simulink model "dinamicaralik"  (R2023b)
settings: Solver=ode45  StartTime=0.0  StopTime=50  FixedStep=0.0001  RelTol=1e-3
InitFcn:
  | Kpz = 0.3 ;
  | KIz = 0;
  | 
  | bh = 0.010290;  % batan hacim m^3
  | m = 10.5     ;  % aracın kütlesi kg
  | g = 9.81     ;  % yer çekimi ivmesi
  | p = 1000     ; % kg / m^3 yogunluk
  | W = m*g      ;  % aracın agırlıgı N
  | B = p*g*bh   ;  % Kaldırma kuvveti  N
  | 
  | xg = 0 ; % rgid body frame e göre ağırlık merkzi kordinatları
  | yg = 0 ;
  | zg = 0.02 ;
  | 
  | Ix = 0.1011 ; % kg *  m ^2
  | Iy = 0.1159 ;
  | Iz = 0.1615 ;
  | 
  | thrustCoefficient = 50/21.5 ;
  | 
  | % Add mass parametreleri
  | Xu_dot = -5.5;   % Surge direction
  | Yv_dot = -12.7;  % Sway direction
  | Zw_dot = -14.57; % Heave direction
  | 
  | Kp_dot = -0.12;  % Roll moment
  | Mq_dot = -0.12;  % Pitch moment
  | Nr_dot = -0.12;  % Yaw moment
  | 
  | % Linear Damping Values (Doğrusal Sönümleme Katsayıları)
  | Xu = -4.03;   % Ns/m
  | Yv = -6.22;   % Ns/m
  | Zw = -5.18;   % Ns/m
  | Kp = -0.07;   % Ns/rad
  | Mq = -0.07;   % Ns/rad
  | Nr = -0.07;   % Ns/rad
  | 
  | % Quadratic Damping Values (Doğrusal Olmayan Sönümleme Katsayıları)
  | Xuu = -18.18;  % Ns^2/m^2
  | Yvv = -21.66;  % Ns^2/m^2
  | Zww = -36.99;  % Ns^2/m^2
  | Kpp = -1.55;   % Ns^2/rad^2
  | Mqq = -1.55;   % Ns^2/rad^2
  | Nrr = -1.55;   % Ns^2/rad^2
undefined symbols (not defined in the file or in its folder): smiData, X, Y, Z
libraries: slpidlib x41, nesl_utility x14, sm_lib x12
(part 6 of 7)

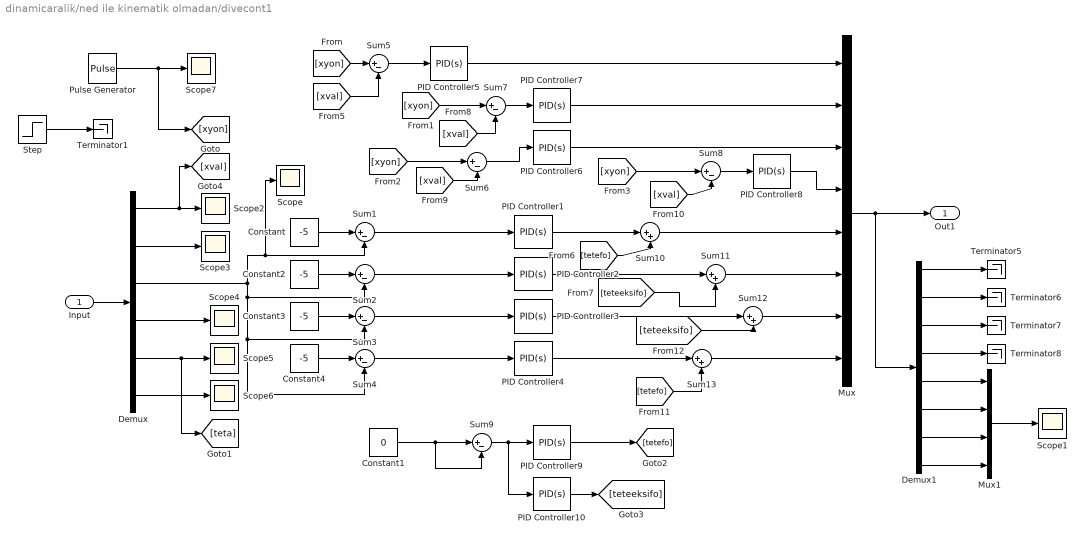
== system dinamicaralik/ned ile kinematik olmadan/divecont1 ==
  Input : Inport
  Constant{,2..4} (4 alike) : Constant  Value=-5
  Constant1 : Constant  Value=0
  Demux : Demux  Outputs=6
  Demux1 : Demux  Outputs=8
  Mux : Mux  Inputs=8
  Mux1 : Mux
  PID Controller1 : slpidlib/PID Controller  Controller=PID  Form=Parallel  TimeDomain=Continuous-time  UseExternalTs=off  SampleTime=-1  IntegratorMethod=Forward Euler  FilterMethod=Forward Euler  ControllerParametersSource=internal  P=Kpz  I=0  UseKiTs=off  D=0  N=100  UseFilter=on  TunerSelectOption=Transfer Function Based (PID Tuner App)  InitialConditionSource=internal  InitialConditionForIntegrator=0  InitialConditionForFilter=0  DifferentiatorICPrevScaledInput=0  ExternalReset=none  TrackingMode=off  Kt=1  LimitOutput=off  SatLimitsSource=internal  UpperSaturationLimit=inf  LowerSaturationLimit=-inf  LinearizeAsGain=on  AntiWindupMode=none  Kb=1  LimitIntegrator=off  UpperIntegratorSaturationLimit=inf  LowerIntegratorSaturationLimit=-inf  POutMin=[]  POutMax=[]  IOutMin=[]  IOutMax=[]  DOutMin=[]  DOutMax=[]  NOutMin=[]  NOutMax=[]  SumOutMin=[]  SumOutMax=[]  SaturationOutMin=[]  SaturationOutMax=[]  PParamMin=[]  PParamMax=[]  IParamMin=[]  IParamMax=[]  DParamMin=[]  DParamMax=[]  NParamMin=[]  NParamMax=[]  KbParamMin=[]  KbParamMax=[]  KtParamMin=[]  KtParamMax=[]  KbOutMin=[]  KbOutMax=[]  KtOutMin=[]  KtOutMax=[]  IntegratorOutMin=[]  IntegratorOutMax=[]  FilterOutMin=[]  FilterOutMax=[]  SumI1OutMin=[]  SumI1OutMax=[]  SumI2OutMin=[]  SumI2OutMax=[]  SumI3OutMin=[]  SumI3OutMax=[]  SumI4OutMin=[]  SumI4OutMax=[]  SumDOutMin=[]  SumDOutMax=[]  DifferentiatorOutMin=[]  DifferentiatorOutMax=[]  FilterDiffOutCoefMin=[]  FilterDiffOutCoefMax=[]  ReciprocalOutMin=[]  ReciprocalOutMax=[]  SumDenOutMin=[]  SumDenOutMax=[]  SumNumOutMin=[]  SumNumOutMax=[]  DivideOutMin=[]  DivideOutMax=[]  UdiffTsProdOutMin=[]  UdiffTsProdOutMax=[]  NTsProdOutMin=[]  NTsProdOutMax=[]  UintegralTsProdOutMin=[]  UintegralTsProdOutMax=[]  UngainTsProdOutMin=[]  UngainTsProdOutMax=[]  ClampingZeroOutDataTypeStr=Inherit: Inherit via back propagation  ClampingZeroOutMin=[]  ClampingZeroOutMax=[]  FilterDenConstantOutDataTypeStr=Inherit: Inherit via back propagation  FilterDenConstantOutMin=[]  FilterDenConstantOutMax=[]  PCopyOutDataTypeStr=Inherit: Inherit via back propagation  PCopyOutMin=[]  PCopyOutMax=[]  NCopyOutDataTypeStr=Inherit: Inherit via back propagation  NCopyOutMin=[]  NCopyOutMax=[]  IntegratorContinuousStateAttributes=''  IntegratorStateMustResolveToSignalObject=off  IntegratorRTWStateStorageClass=Auto  FilterContinuousStateAttributes=''  FilterStateMustResolveToSignalObject=off  FilterRTWStateStorageClass=Auto  ParallelPVariant=InternalParameters  IdealPVariant=Disabled  IVariant=InternalParameters  DVariant=InternalParameters  IntegratorVariant=Continuous  SatVariant=Disabled  AWVariant=Passthrough  PCopyVariant=Disabled  TRVariant=Disabled  FdbkBlocksVariant=Forward  IdealPFdbkVariant=Disabled  SatFdbkVariant=Disabled  DerivativeFilterVariant=ContFilter  NVariant=InternalParameters  NCopyVariant=Disabled  FilterICVariant=InternalICsFilter  IntegratorICVariant=InternalICs  ExternalResetVariant=Disabled  TRSumVariant=Passthrough  SumFdbkVariant=Disabled  SumVariant=Sum_PID  TsampFilterVariant=InternalTs  TsampNgainVariant=Passthrough  TsampIntegralVariant=Disabled_SignalSpec  ExternalSaturationOutDataTypeStr=Inherit: Same as second input
  PID Controller10 : slpidlib/PID Controller  Controller=PID  Form=Parallel  TimeDomain=Continuous-time  UseExternalTs=off  SampleTime=-1  IntegratorMethod=Forward Euler  FilterMethod=Forward Euler  ControllerParametersSource=internal  P=-0.1  I=0  UseKiTs=off  D=0  N=100  UseFilter=on  TunerSelectOption=Transfer Function Based (PID Tuner App)  InitialConditionSource=internal  InitialConditionForIntegrator=0  InitialConditionForFilter=0  DifferentiatorICPrevScaledInput=0  ExternalReset=none  TrackingMode=off  Kt=1  LimitOutput=off  SatLimitsSource=internal  UpperSaturationLimit=inf  LowerSaturationLimit=-inf  LinearizeAsGain=on  AntiWindupMode=none  Kb=1  LimitIntegrator=off  UpperIntegratorSaturationLimit=inf  LowerIntegratorSaturationLimit=-inf  POutMin=[]  POutMax=[]  IOutMin=[]  IOutMax=[]  DOutMin=[]  DOutMax=[]  NOutMin=[]  NOutMax=[]  SumOutMin=[]  SumOutMax=[]  SaturationOutMin=[]  SaturationOutMax=[]  PParamMin=[]  PParamMax=[]  IParamMin=[]  IParamMax=[]  DParamMin=[]  DParamMax=[]  NParamMin=[]  NParamMax=[]  KbParamMin=[]  KbParamMax=[]  KtParamMin=[]  KtParamMax=[]  KbOutMin=[]  KbOutMax=[]  KtOutMin=[]  KtOutMax=[]  IntegratorOutMin=[]  IntegratorOutMax=[]  FilterOutMin=[]  FilterOutMax=[]  SumI1OutMin=[]  SumI1OutMax=[]  SumI2OutMin=[]  SumI2OutMax=[]  SumI3OutMin=[]  SumI3OutMax=[]  SumI4OutMin=[]  SumI4OutMax=[]  SumDOutMin=[]  SumDOutMax=[]  DifferentiatorOutMin=[]  DifferentiatorOutMax=[]  FilterDiffOutCoefMin=[]  FilterDiffOutCoefMax=[]  ReciprocalOutMin=[]  ReciprocalOutMax=[]  SumDenOutMin=[]  SumDenOutMax=[]  SumNumOutMin=[]  SumNumOutMax=[]  DivideOutMin=[]  DivideOutMax=[]  UdiffTsProdOutMin=[]  UdiffTsProdOutMax=[]  NTsProdOutMin=[]  NTsProdOutMax=[]  UintegralTsProdOutMin=[]  UintegralTsProdOutMax=[]  UngainTsProdOutMin=[]  UngainTsProdOutMax=[]  ClampingZeroOutDataTypeStr=Inherit: Inherit via back propagation  ClampingZeroOutMin=[]  ClampingZeroOutMax=[]  FilterDenConstantOutDataTypeStr=Inherit: Inherit via back propagation  FilterDenConstantOutMin=[]  FilterDenConstantOutMax=[]  PCopyOutDataTypeStr=Inherit: Inherit via back propagation  PCopyOutMin=[]  PCopyOutMax=[]  NCopyOutDataTypeStr=Inherit: Inherit via back propagation  NCopyOutMin=[]  NCopyOutMax=[]  IntegratorContinuousStateAttributes=''  IntegratorStateMustResolveToSignalObject=off  IntegratorRTWStateStorageClass=Auto  FilterContinuousStateAttributes=''  FilterStateMustResolveToSignalObject=off  FilterRTWStateStorageClass=Auto  ParallelPVariant=InternalParameters  IdealPVariant=Disabled  IVariant=InternalParameters  DVariant=InternalParameters  IntegratorVariant=Continuous  SatVariant=Disabled  AWVariant=Passthrough  PCopyVariant=Disabled  TRVariant=Disabled  FdbkBlocksVariant=Forward  IdealPFdbkVariant=Disabled  SatFdbkVariant=Disabled  DerivativeFilterVariant=ContFilter  NVariant=InternalParameters  NCopyVariant=Disabled  FilterICVariant=InternalICsFilter  IntegratorICVariant=InternalICs  ExternalResetVariant=Disabled  TRSumVariant=Passthrough  SumFdbkVariant=Disabled  SumVariant=Sum_PID  TsampFilterVariant=InternalTs  TsampNgainVariant=Passthrough  TsampIntegralVariant=Disabled_SignalSpec  ExternalSaturationOutDataTypeStr=Inherit: Same as second input
  PID Controller2 : slpidlib/PID Controller  Controller=PID  Form=Parallel  TimeDomain=Continuous-time  UseExternalTs=off  SampleTime=-1  IntegratorMethod=Forward Euler  FilterMethod=Forward Euler  ControllerParametersSource=internal  P=-Kpz  I=0  UseKiTs=off  D=0  N=100  UseFilter=on  TunerSelectOption=Transfer Function Based (PID Tuner App)  InitialConditionSource=internal  InitialConditionForIntegrator=0  InitialConditionForFilter=0  DifferentiatorICPrevScaledInput=0  ExternalReset=none  TrackingMode=off  Kt=1  LimitOutput=off  SatLimitsSource=internal  UpperSaturationLimit=inf  LowerSaturationLimit=-inf  LinearizeAsGain=on  AntiWindupMode=none  Kb=1  LimitIntegrator=off  UpperIntegratorSaturationLimit=inf  LowerIntegratorSaturationLimit=-inf  POutMin=[]  POutMax=[]  IOutMin=[]  IOutMax=[]  DOutMin=[]  DOutMax=[]  NOutMin=[]  NOutMax=[]  SumOutMin=[]  SumOutMax=[]  SaturationOutMin=[]  SaturationOutMax=[]  PParamMin=[]  PParamMax=[]  IParamMin=[]  IParamMax=[]  DParamMin=[]  DParamMax=[]  NParamMin=[]  NParamMax=[]  KbParamMin=[]  KbParamMax=[]  KtParamMin=[]  KtParamMax=[]  KbOutMin=[]  KbOutMax=[]  KtOutMin=[]  KtOutMax=[]  IntegratorOutMin=[]  IntegratorOutMax=[]  FilterOutMin=[]  FilterOutMax=[]  SumI1OutMin=[]  SumI1OutMax=[]  SumI2OutMin=[]  SumI2OutMax=[]  SumI3OutMin=[]  SumI3OutMax=[]  SumI4OutMin=[]  SumI4OutMax=[]  SumDOutMin=[]  SumDOutMax=[]  DifferentiatorOutMin=[]  DifferentiatorOutMax=[]  FilterDiffOutCoefMin=[]  FilterDiffOutCoefMax=[]  ReciprocalOutMin=[]  ReciprocalOutMax=[]  SumDenOutMin=[]  SumDenOutMax=[]  SumNumOutMin=[]  SumNumOutMax=[]  DivideOutMin=[]  DivideOutMax=[]  UdiffTsProdOutMin=[]  UdiffTsProdOutMax=[]  NTsProdOutMin=[]  NTsProdOutMax=[]  UintegralTsProdOutMin=[]  UintegralTsProdOutMax=[]  UngainTsProdOutMin=[]  UngainTsProdOutMax=[]  ClampingZeroOutDataTypeStr=Inherit: Inherit via back propagation  ClampingZeroOutMin=[]  ClampingZeroOutMax=[]  FilterDenConstantOutDataTypeStr=Inherit: Inherit via back propagation  FilterDenConstantOutMin=[]  FilterDenConstantOutMax=[]  PCopyOutDataTypeStr=Inherit: Inherit via back propagation  PCopyOutMin=[]  PCopyOutMax=[]  NCopyOutDataTypeStr=Inherit: Inherit via back propagation  NCopyOutMin=[]  NCopyOutMax=[]  IntegratorContinuousStateAttributes=''  IntegratorStateMustResolveToSignalObject=off  IntegratorRTWStateStorageClass=Auto  FilterContinuousStateAttributes=''  FilterStateMustResolveToSignalObject=off  FilterRTWStateStorageClass=Auto  ParallelPVariant=InternalParameters  IdealPVariant=Disabled  IVariant=InternalParameters  DVariant=InternalParameters  IntegratorVariant=Continuous  SatVariant=Disabled  AWVariant=Passthrough  PCopyVariant=Disabled  TRVariant=Disabled  FdbkBlocksVariant=Forward  IdealPFdbkVariant=Disabled  SatFdbkVariant=Disabled  DerivativeFilterVariant=ContFilter  NVariant=InternalParameters  NCopyVariant=Disabled  FilterICVariant=InternalICsFilter  IntegratorICVariant=InternalICs  ExternalResetVariant=Disabled  TRSumVariant=Passthrough  SumFdbkVariant=Disabled  SumVariant=Sum_PID  TsampFilterVariant=InternalTs  TsampNgainVariant=Passthrough  TsampIntegralVariant=Disabled_SignalSpec  ExternalSaturationOutDataTypeStr=Inherit: Same as second input
  PID Controller3 : slpidlib/PID Controller  Controller=PID  Form=Parallel  TimeDomain=Continuous-time  UseExternalTs=off  SampleTime=-1  IntegratorMethod=Forward Euler  FilterMethod=Forward Euler  ControllerParametersSource=internal  P=-Kpz  I=0  UseKiTs=off  D=0  N=100  UseFilter=on  TunerSelectOption=Transfer Function Based (PID Tuner App)  InitialConditionSource=internal  InitialConditionForIntegrator=0  InitialConditionForFilter=0  DifferentiatorICPrevScaledInput=0  ExternalReset=none  TrackingMode=off  Kt=1  LimitOutput=off  SatLimitsSource=internal  UpperSaturationLimit=inf  LowerSaturationLimit=-inf  LinearizeAsGain=on  AntiWindupMode=none  Kb=1  LimitIntegrator=off  UpperIntegratorSaturationLimit=inf  LowerIntegratorSaturationLimit=-inf  POutMin=[]  POutMax=[]  IOutMin=[]  IOutMax=[]  DOutMin=[]  DOutMax=[]  NOutMin=[]  NOutMax=[]  SumOutMin=[]  SumOutMax=[]  SaturationOutMin=[]  SaturationOutMax=[]  PParamMin=[]  PParamMax=[]  IParamMin=[]  IParamMax=[]  DParamMin=[]  DParamMax=[]  NParamMin=[]  NParamMax=[]  KbParamMin=[]  KbParamMax=[]  KtParamMin=[]  KtParamMax=[]  KbOutMin=[]  KbOutMax=[]  KtOutMin=[]  KtOutMax=[]  IntegratorOutMin=[]  IntegratorOutMax=[]  FilterOutMin=[]  FilterOutMax=[]  SumI1OutMin=[]  SumI1OutMax=[]  SumI2OutMin=[]  SumI2OutMax=[]  SumI3OutMin=[]  SumI3OutMax=[]  SumI4OutMin=[]  SumI4OutMax=[]  SumDOutMin=[]  SumDOutMax=[]  DifferentiatorOutMin=[]  DifferentiatorOutMax=[]  FilterDiffOutCoefMin=[]  FilterDiffOutCoefMax=[]  ReciprocalOutMin=[]  ReciprocalOutMax=[]  SumDenOutMin=[]  SumDenOutMax=[]  SumNumOutMin=[]  SumNumOutMax=[]  DivideOutMin=[]  DivideOutMax=[]  UdiffTsProdOutMin=[]  UdiffTsProdOutMax=[]  NTsProdOutMin=[]  NTsProdOutMax=[]  UintegralTsProdOutMin=[]  UintegralTsProdOutMax=[]  UngainTsProdOutMin=[]  UngainTsProdOutMax=[]  ClampingZeroOutDataTypeStr=Inherit: Inherit via back propagation  ClampingZeroOutMin=[]  ClampingZeroOutMax=[]  FilterDenConstantOutDataTypeStr=Inherit: Inherit via back propagation  FilterDenConstantOutMin=[]  FilterDenConstantOutMax=[]  PCopyOutDataTypeStr=Inherit: Inherit via back propagation  PCopyOutMin=[]  PCopyOutMax=[]  NCopyOutDataTypeStr=Inherit: Inherit via back propagation  NCopyOutMin=[]  NCopyOutMax=[]  IntegratorContinuousStateAttributes=''  IntegratorStateMustResolveToSignalObject=off  IntegratorRTWStateStorageClass=Auto  FilterContinuousStateAttributes=''  FilterStateMustResolveToSignalObject=off  FilterRTWStateStorageClass=Auto  ParallelPVariant=InternalParameters  IdealPVariant=Disabled  IVariant=InternalParameters  DVariant=InternalParameters  IntegratorVariant=Continuous  SatVariant=Disabled  AWVariant=Passthrough  PCopyVariant=Disabled  TRVariant=Disabled  FdbkBlocksVariant=Forward  IdealPFdbkVariant=Disabled  SatFdbkVariant=Disabled  DerivativeFilterVariant=ContFilter  NVariant=InternalParameters  NCopyVariant=Disabled  FilterICVariant=InternalICsFilter  IntegratorICVariant=InternalICs  ExternalResetVariant=Disabled  TRSumVariant=Passthrough  SumFdbkVariant=Disabled  SumVariant=Sum_PID  TsampFilterVariant=InternalTs  TsampNgainVariant=Passthrough  TsampIntegralVariant=Disabled_SignalSpec  ExternalSaturationOutDataTypeStr=Inherit: Same as second input
  PID Controller4 : slpidlib/PID Controller  Controller=PID  Form=Parallel  TimeDomain=Continuous-time  UseExternalTs=off  SampleTime=-1  IntegratorMethod=Forward Euler  FilterMethod=Forward Euler  ControllerParametersSource=internal  P=Kpz  I=0  UseKiTs=off  D=0  N=100  UseFilter=on  TunerSelectOption=Transfer Function Based (PID Tuner App)  InitialConditionSource=internal  InitialConditionForIntegrator=0  InitialConditionForFilter=0  DifferentiatorICPrevScaledInput=0  ExternalReset=none  TrackingMode=off  Kt=1  LimitOutput=off  SatLimitsSource=internal  UpperSaturationLimit=inf  LowerSaturationLimit=-inf  LinearizeAsGain=on  AntiWindupMode=none  Kb=1  LimitIntegrator=off  UpperIntegratorSaturationLimit=inf  LowerIntegratorSaturationLimit=-inf  POutMin=[]  POutMax=[]  IOutMin=[]  IOutMax=[]  DOutMin=[]  DOutMax=[]  NOutMin=[]  NOutMax=[]  SumOutMin=[]  SumOutMax=[]  SaturationOutMin=[]  SaturationOutMax=[]  PParamMin=[]  PParamMax=[]  IParamMin=[]  IParamMax=[]  DParamMin=[]  DParamMax=[]  NParamMin=[]  NParamMax=[]  KbParamMin=[]  KbParamMax=[]  KtParamMin=[]  KtParamMax=[]  KbOutMin=[]  KbOutMax=[]  KtOutMin=[]  KtOutMax=[]  IntegratorOutMin=[]  IntegratorOutMax=[]  FilterOutMin=[]  FilterOutMax=[]  SumI1OutMin=[]  SumI1OutMax=[]  SumI2OutMin=[]  SumI2OutMax=[]  SumI3OutMin=[]  SumI3OutMax=[]  SumI4OutMin=[]  SumI4OutMax=[]  SumDOutMin=[]  SumDOutMax=[]  DifferentiatorOutMin=[]  DifferentiatorOutMax=[]  FilterDiffOutCoefMin=[]  FilterDiffOutCoefMax=[]  ReciprocalOutMin=[]  ReciprocalOutMax=[]  SumDenOutMin=[]  SumDenOutMax=[]  SumNumOutMin=[]  SumNumOutMax=[]  DivideOutMin=[]  DivideOutMax=[]  UdiffTsProdOutMin=[]  UdiffTsProdOutMax=[]  NTsProdOutMin=[]  NTsProdOutMax=[]  UintegralTsProdOutMin=[]  UintegralTsProdOutMax=[]  UngainTsProdOutMin=[]  UngainTsProdOutMax=[]  ClampingZeroOutDataTypeStr=Inherit: Inherit via back propagation  ClampingZeroOutMin=[]  ClampingZeroOutMax=[]  FilterDenConstantOutDataTypeStr=Inherit: Inherit via back propagation  FilterDenConstantOutMin=[]  FilterDenConstantOutMax=[]  PCopyOutDataTypeStr=Inherit: Inherit via back propagation  PCopyOutMin=[]  PCopyOutMax=[]  NCopyOutDataTypeStr=Inherit: Inherit via back propagation  NCopyOutMin=[]  NCopyOutMax=[]  IntegratorContinuousStateAttributes=''  IntegratorStateMustResolveToSignalObject=off  IntegratorRTWStateStorageClass=Auto  FilterContinuousStateAttributes=''  FilterStateMustResolveToSignalObject=off  FilterRTWStateStorageClass=Auto  ParallelPVariant=InternalParameters  IdealPVariant=Disabled  IVariant=InternalParameters  DVariant=InternalParameters  IntegratorVariant=Continuous  SatVariant=Disabled  AWVariant=Passthrough  PCopyVariant=Disabled  TRVariant=Disabled  FdbkBlocksVariant=Forward  IdealPFdbkVariant=Disabled  SatFdbkVariant=Disabled  DerivativeFilterVariant=ContFilter  NVariant=InternalParameters  NCopyVariant=Disabled  FilterICVariant=InternalICsFilter  IntegratorICVariant=InternalICs  ExternalResetVariant=Disabled  TRSumVariant=Passthrough  SumFdbkVariant=Disabled  SumVariant=Sum_PID  TsampFilterVariant=InternalTs  TsampNgainVariant=Passthrough  TsampIntegralVariant=Disabled_SignalSpec  ExternalSaturationOutDataTypeStr=Inherit: Same as second input
  PID Controller5 : slpidlib/PID Controller  Controller=PID  Form=Parallel  TimeDomain=Continuous-time  UseExternalTs=off  SampleTime=-1  IntegratorMethod=Forward Euler  FilterMethod=Forward Euler  ControllerParametersSource=internal  P=Kpz  I=KIz  UseKiTs=off  D=0  N=100  UseFilter=on  TunerSelectOption=Transfer Function Based (PID Tuner App)  InitialConditionSource=internal  InitialConditionForIntegrator=0  InitialConditionForFilter=0  DifferentiatorICPrevScaledInput=0  ExternalReset=none  TrackingMode=off  Kt=1  LimitOutput=off  SatLimitsSource=internal  UpperSaturationLimit=inf  LowerSaturationLimit=-inf  LinearizeAsGain=on  AntiWindupMode=none  Kb=1  LimitIntegrator=off  UpperIntegratorSaturationLimit=inf  LowerIntegratorSaturationLimit=-inf  POutMin=[]  POutMax=[]  IOutMin=[]  IOutMax=[]  DOutMin=[]  DOutMax=[]  NOutMin=[]  NOutMax=[]  SumOutMin=[]  SumOutMax=[]  SaturationOutMin=[]  SaturationOutMax=[]  PParamMin=[]  PParamMax=[]  IParamMin=[]  IParamMax=[]  DParamMin=[]  DParamMax=[]  NParamMin=[]  NParamMax=[]  KbParamMin=[]  KbParamMax=[]  KtParamMin=[]  KtParamMax=[]  KbOutMin=[]  KbOutMax=[]  KtOutMin=[]  KtOutMax=[]  IntegratorOutMin=[]  IntegratorOutMax=[]  FilterOutMin=[]  FilterOutMax=[]  SumI1OutMin=[]  SumI1OutMax=[]  SumI2OutMin=[]  SumI2OutMax=[]  SumI3OutMin=[]  SumI3OutMax=[]  SumI4OutMin=[]  SumI4OutMax=[]  SumDOutMin=[]  SumDOutMax=[]  DifferentiatorOutMin=[]  DifferentiatorOutMax=[]  FilterDiffOutCoefMin=[]  FilterDiffOutCoefMax=[]  ReciprocalOutMin=[]  ReciprocalOutMax=[]  SumDenOutMin=[]  SumDenOutMax=[]  SumNumOutMin=[]  SumNumOutMax=[]  DivideOutMin=[]  DivideOutMax=[]  UdiffTsProdOutMin=[]  UdiffTsProdOutMax=[]  NTsProdOutMin=[]  NTsProdOutMax=[]  UintegralTsProdOutMin=[]  UintegralTsProdOutMax=[]  UngainTsProdOutMin=[]  UngainTsProdOutMax=[]  ClampingZeroOutDataTypeStr=Inherit: Inherit via back propagation  ClampingZeroOutMin=[]  ClampingZeroOutMax=[]  FilterDenConstantOutDataTypeStr=Inherit: Inherit via back propagation  FilterDenConstantOutMin=[]  FilterDenConstantOutMax=[]  PCopyOutDataTypeStr=Inherit: Inherit via back propagation  PCopyOutMin=[]  PCopyOutMax=[]  NCopyOutDataTypeStr=Inherit: Inherit via back propagation  NCopyOutMin=[]  NCopyOutMax=[]  IntegratorContinuousStateAttributes=''  IntegratorStateMustResolveToSignalObject=off  IntegratorRTWStateStorageClass=Auto  FilterContinuousStateAttributes=''  FilterStateMustResolveToSignalObject=off  FilterRTWStateStorageClass=Auto  ParallelPVariant=InternalParameters  IdealPVariant=Disabled  IVariant=InternalParameters  DVariant=InternalParameters  IntegratorVariant=Continuous  SatVariant=Disabled  AWVariant=Passthrough  PCopyVariant=Disabled  TRVariant=Disabled  FdbkBlocksVariant=Forward  IdealPFdbkVariant=Disabled  SatFdbkVariant=Disabled  DerivativeFilterVariant=ContFilter  NVariant=InternalParameters  NCopyVariant=Disabled  FilterICVariant=InternalICsFilter  IntegratorICVariant=InternalICs  ExternalResetVariant=Disabled  TRSumVariant=Passthrough  SumFdbkVariant=Disabled  SumVariant=Sum_PID  TsampFilterVariant=InternalTs  TsampNgainVariant=Passthrough  TsampIntegralVariant=Disabled_SignalSpec  ExternalSaturationOutDataTypeStr=Inherit: Same as second input
  PID Controller6 : slpidlib/PID Controller  Controller=PID  Form=Parallel  TimeDomain=Continuous-time  UseExternalTs=off  SampleTime=-1  IntegratorMethod=Forward Euler  FilterMethod=Forward Euler  ControllerParametersSource=internal  P=-Kpz  I=KIz  UseKiTs=off  D=0  N=100  UseFilter=on  TunerSelectOption=Transfer Function Based (PID Tuner App)  InitialConditionSource=internal  InitialConditionForIntegrator=0  InitialConditionForFilter=0  DifferentiatorICPrevScaledInput=0  ExternalReset=none  TrackingMode=off  Kt=1  LimitOutput=off  SatLimitsSource=internal  UpperSaturationLimit=inf  LowerSaturationLimit=-inf  LinearizeAsGain=on  AntiWindupMode=none  Kb=1  LimitIntegrator=off  UpperIntegratorSaturationLimit=inf  LowerIntegratorSaturationLimit=-inf  POutMin=[]  POutMax=[]  IOutMin=[]  IOutMax=[]  DOutMin=[]  DOutMax=[]  NOutMin=[]  NOutMax=[]  SumOutMin=[]  SumOutMax=[]  SaturationOutMin=[]  SaturationOutMax=[]  PParamMin=[]  PParamMax=[]  IParamMin=[]  IParamMax=[]  DParamMin=[]  DParamMax=[]  NParamMin=[]  NParamMax=[]  KbParamMin=[]  KbParamMax=[]  KtParamMin=[]  KtParamMax=[]  KbOutMin=[]  KbOutMax=[]  KtOutMin=[]  KtOutMax=[]  IntegratorOutMin=[]  IntegratorOutMax=[]  FilterOutMin=[]  FilterOutMax=[]  SumI1OutMin=[]  SumI1OutMax=[]  SumI2OutMin=[]  SumI2OutMax=[]  SumI3OutMin=[]  SumI3OutMax=[]  SumI4OutMin=[]  SumI4OutMax=[]  SumDOutMin=[]  SumDOutMax=[]  DifferentiatorOutMin=[]  DifferentiatorOutMax=[]  FilterDiffOutCoefMin=[]  FilterDiffOutCoefMax=[]  ReciprocalOutMin=[]  ReciprocalOutMax=[]  SumDenOutMin=[]  SumDenOutMax=[]  SumNumOutMin=[]  SumNumOutMax=[]  DivideOutMin=[]  DivideOutMax=[]  UdiffTsProdOutMin=[]  UdiffTsProdOutMax=[]  NTsProdOutMin=[]  NTsProdOutMax=[]  UintegralTsProdOutMin=[]  UintegralTsProdOutMax=[]  UngainTsProdOutMin=[]  UngainTsProdOutMax=[]  ClampingZeroOutDataTypeStr=Inherit: Inherit via back propagation  ClampingZeroOutMin=[]  ClampingZeroOutMax=[]  FilterDenConstantOutDataTypeStr=Inherit: Inherit via back propagation  FilterDenConstantOutMin=[]  FilterDenConstantOutMax=[]  PCopyOutDataTypeStr=Inherit: Inherit via back propagation  PCopyOutMin=[]  PCopyOutMax=[]  NCopyOutDataTypeStr=Inherit: Inherit via back propagation  NCopyOutMin=[]  NCopyOutMax=[]  IntegratorContinuousStateAttributes=''  IntegratorStateMustResolveToSignalObject=off  IntegratorRTWStateStorageClass=Auto  FilterContinuousStateAttributes=''  FilterStateMustResolveToSignalObject=off  FilterRTWStateStorageClass=Auto  ParallelPVariant=InternalParameters  IdealPVariant=Disabled  IVariant=InternalParameters  DVariant=InternalParameters  IntegratorVariant=Continuous  SatVariant=Disabled  AWVariant=Passthrough  PCopyVariant=Disabled  TRVariant=Disabled  FdbkBlocksVariant=Forward  IdealPFdbkVariant=Disabled  SatFdbkVariant=Disabled  DerivativeFilterVariant=ContFilter  NVariant=InternalParameters  NCopyVariant=Disabled  FilterICVariant=InternalICsFilter  IntegratorICVariant=InternalICs  ExternalResetVariant=Disabled  TRSumVariant=Passthrough  SumFdbkVariant=Disabled  SumVariant=Sum_PID  TsampFilterVariant=InternalTs  TsampNgainVariant=Passthrough  TsampIntegralVariant=Disabled_SignalSpec  ExternalSaturationOutDataTypeStr=Inherit: Same as second input
  PID Controller7 : slpidlib/PID Controller  Controller=PID  Form=Parallel  TimeDomain=Continuous-time  UseExternalTs=off  SampleTime=-1  IntegratorMethod=Forward Euler  FilterMethod=Forward Euler  ControllerParametersSource=internal  P=Kpz  I=KIz  UseKiTs=off  D=0  N=100  UseFilter=on  TunerSelectOption=Transfer Function Based (PID Tuner App)  InitialConditionSource=internal  InitialConditionForIntegrator=0  InitialConditionForFilter=0  DifferentiatorICPrevScaledInput=0  ExternalReset=none  TrackingMode=off  Kt=1  LimitOutput=off  SatLimitsSource=internal  UpperSaturationLimit=inf  LowerSaturationLimit=-inf  LinearizeAsGain=on  AntiWindupMode=none  Kb=1  LimitIntegrator=off  UpperIntegratorSaturationLimit=inf  LowerIntegratorSaturationLimit=-inf  POutMin=[]  POutMax=[]  IOutMin=[]  IOutMax=[]  DOutMin=[]  DOutMax=[]  NOutMin=[]  NOutMax=[]  SumOutMin=[]  SumOutMax=[]  SaturationOutMin=[]  SaturationOutMax=[]  PParamMin=[]  PParamMax=[]  IParamMin=[]  IParamMax=[]  DParamMin=[]  DParamMax=[]  NParamMin=[]  NParamMax=[]  KbParamMin=[]  KbParamMax=[]  KtParamMin=[]  KtParamMax=[]  KbOutMin=[]  KbOutMax=[]  KtOutMin=[]  KtOutMax=[]  IntegratorOutMin=[]  IntegratorOutMax=[]  FilterOutMin=[]  FilterOutMax=[]  SumI1OutMin=[]  SumI1OutMax=[]  SumI2OutMin=[]  SumI2OutMax=[]  SumI3OutMin=[]  SumI3OutMax=[]  SumI4OutMin=[]  SumI4OutMax=[]  SumDOutMin=[]  SumDOutMax=[]  DifferentiatorOutMin=[]  DifferentiatorOutMax=[]  FilterDiffOutCoefMin=[]  FilterDiffOutCoefMax=[]  ReciprocalOutMin=[]  ReciprocalOutMax=[]  SumDenOutMin=[]  SumDenOutMax=[]  SumNumOutMin=[]  SumNumOutMax=[]  DivideOutMin=[]  DivideOutMax=[]  UdiffTsProdOutMin=[]  UdiffTsProdOutMax=[]  NTsProdOutMin=[]  NTsProdOutMax=[]  UintegralTsProdOutMin=[]  UintegralTsProdOutMax=[]  UngainTsProdOutMin=[]  UngainTsProdOutMax=[]  ClampingZeroOutDataTypeStr=Inherit: Inherit via back propagation  ClampingZeroOutMin=[]  ClampingZeroOutMax=[]  FilterDenConstantOutDataTypeStr=Inherit: Inherit via back propagation  FilterDenConstantOutMin=[]  FilterDenConstantOutMax=[]  PCopyOutDataTypeStr=Inherit: Inherit via back propagation  PCopyOutMin=[]  PCopyOutMax=[]  NCopyOutDataTypeStr=Inherit: Inherit via back propagation  NCopyOutMin=[]  NCopyOutMax=[]  IntegratorContinuousStateAttributes=''  IntegratorStateMustResolveToSignalObject=off  IntegratorRTWStateStorageClass=Auto  FilterContinuousStateAttributes=''  FilterStateMustResolveToSignalObject=off  FilterRTWStateStorageClass=Auto  ParallelPVariant=InternalParameters  IdealPVariant=Disabled  IVariant=InternalParameters  DVariant=InternalParameters  IntegratorVariant=Continuous  SatVariant=Disabled  AWVariant=Passthrough  PCopyVariant=Disabled  TRVariant=Disabled  FdbkBlocksVariant=Forward  IdealPFdbkVariant=Disabled  SatFdbkVariant=Disabled  DerivativeFilterVariant=ContFilter  NVariant=InternalParameters  NCopyVariant=Disabled  FilterICVariant=InternalICsFilter  IntegratorICVariant=InternalICs  ExternalResetVariant=Disabled  TRSumVariant=Passthrough  SumFdbkVariant=Disabled  SumVariant=Sum_PID  TsampFilterVariant=InternalTs  TsampNgainVariant=Passthrough  TsampIntegralVariant=Disabled_SignalSpec  ExternalSaturationOutDataTypeStr=Inherit: Same as second input
  PID Controller8 : slpidlib/PID Controller  Controller=PID  Form=Parallel  TimeDomain=Continuous-time  UseExternalTs=off  SampleTime=-1  IntegratorMethod=Forward Euler  FilterMethod=Forward Euler  ControllerParametersSource=internal  P=-Kpz  I=KIz  UseKiTs=off  D=0  N=100  UseFilter=on  TunerSelectOption=Transfer Function Based (PID Tuner App)  InitialConditionSource=internal  InitialConditionForIntegrator=0  InitialConditionForFilter=0  DifferentiatorICPrevScaledInput=0  ExternalReset=none  TrackingMode=off  Kt=1  LimitOutput=off  SatLimitsSource=internal  UpperSaturationLimit=inf  LowerSaturationLimit=-inf  LinearizeAsGain=on  AntiWindupMode=none  Kb=1  LimitIntegrator=off  UpperIntegratorSaturationLimit=inf  LowerIntegratorSaturationLimit=-inf  POutMin=[]  POutMax=[]  IOutMin=[]  IOutMax=[]  DOutMin=[]  DOutMax=[]  NOutMin=[]  NOutMax=[]  SumOutMin=[]  SumOutMax=[]  SaturationOutMin=[]  SaturationOutMax=[]  PParamMin=[]  PParamMax=[]  IParamMin=[]  IParamMax=[]  DParamMin=[]  DParamMax=[]  NParamMin=[]  NParamMax=[]  KbParamMin=[]  KbParamMax=[]  KtParamMin=[]  KtParamMax=[]  KbOutMin=[]  KbOutMax=[]  KtOutMin=[]  KtOutMax=[]  IntegratorOutMin=[]  IntegratorOutMax=[]  FilterOutMin=[]  FilterOutMax=[]  SumI1OutMin=[]  SumI1OutMax=[]  SumI2OutMin=[]  SumI2OutMax=[]  SumI3OutMin=[]  SumI3OutMax=[]  SumI4OutMin=[]  SumI4OutMax=[]  SumDOutMin=[]  SumDOutMax=[]  DifferentiatorOutMin=[]  DifferentiatorOutMax=[]  FilterDiffOutCoefMin=[]  FilterDiffOutCoefMax=[]  ReciprocalOutMin=[]  ReciprocalOutMax=[]  SumDenOutMin=[]  SumDenOutMax=[]  SumNumOutMin=[]  SumNumOutMax=[]  DivideOutMin=[]  DivideOutMax=[]  UdiffTsProdOutMin=[]  UdiffTsProdOutMax=[]  NTsProdOutMin=[]  NTsProdOutMax=[]  UintegralTsProdOutMin=[]  UintegralTsProdOutMax=[]  UngainTsProdOutMin=[]  UngainTsProdOutMax=[]  ClampingZeroOutDataTypeStr=Inherit: Inherit via back propagation  ClampingZeroOutMin=[]  ClampingZeroOutMax=[]  FilterDenConstantOutDataTypeStr=Inherit: Inherit via back propagation  FilterDenConstantOutMin=[]  FilterDenConstantOutMax=[]  PCopyOutDataTypeStr=Inherit: Inherit via back propagation  PCopyOutMin=[]  PCopyOutMax=[]  NCopyOutDataTypeStr=Inherit: Inherit via back propagation  NCopyOutMin=[]  NCopyOutMax=[]  IntegratorContinuousStateAttributes=''  IntegratorStateMustResolveToSignalObject=off  IntegratorRTWStateStorageClass=Auto  FilterContinuousStateAttributes=''  FilterStateMustResolveToSignalObject=off  FilterRTWStateStorageClass=Auto  ParallelPVariant=InternalParameters  IdealPVariant=Disabled  IVariant=InternalParameters  DVariant=InternalParameters  IntegratorVariant=Continuous  SatVariant=Disabled  AWVariant=Passthrough  PCopyVariant=Disabled  TRVariant=Disabled  FdbkBlocksVariant=Forward  IdealPFdbkVariant=Disabled  SatFdbkVariant=Disabled  DerivativeFilterVariant=ContFilter  NVariant=InternalParameters  NCopyVariant=Disabled  FilterICVariant=InternalICsFilter  IntegratorICVariant=InternalICs  ExternalResetVariant=Disabled  TRSumVariant=Passthrough  SumFdbkVariant=Disabled  SumVariant=Sum_PID  TsampFilterVariant=InternalTs  TsampNgainVariant=Passthrough  TsampIntegralVariant=Disabled_SignalSpec  ExternalSaturationOutDataTypeStr=Inherit: Same as second input
  PID Controller9 : slpidlib/PID Controller  Controller=PID  Form=Parallel  TimeDomain=Continuous-time  UseExternalTs=off  SampleTime=-1  IntegratorMethod=Forward Euler  FilterMethod=Forward Euler  ControllerParametersSource=internal  P=0.1  I=0  UseKiTs=off  D=0  N=100  UseFilter=on  TunerSelectOption=Transfer Function Based (PID Tuner App)  InitialConditionSource=internal  InitialConditionForIntegrator=0  InitialConditionForFilter=0  DifferentiatorICPrevScaledInput=0  ExternalReset=none  TrackingMode=off  Kt=1  LimitOutput=off  SatLimitsSource=internal  UpperSaturationLimit=inf  LowerSaturationLimit=-inf  LinearizeAsGain=on  AntiWindupMode=none  Kb=1  LimitIntegrator=off  UpperIntegratorSaturationLimit=inf  LowerIntegratorSaturationLimit=-inf  POutMin=[]  POutMax=[]  IOutMin=[]  IOutMax=[]  DOutMin=[]  DOutMax=[]  NOutMin=[]  NOutMax=[]  SumOutMin=[]  SumOutMax=[]  SaturationOutMin=[]  SaturationOutMax=[]  PParamMin=[]  PParamMax=[]  IParamMin=[]  IParamMax=[]  DParamMin=[]  DParamMax=[]  NParamMin=[]  NParamMax=[]  KbParamMin=[]  KbParamMax=[]  KtParamMin=[]  KtParamMax=[]  KbOutMin=[]  KbOutMax=[]  KtOutMin=[]  KtOutMax=[]  IntegratorOutMin=[]  IntegratorOutMax=[]  FilterOutMin=[]  FilterOutMax=[]  SumI1OutMin=[]  SumI1OutMax=[]  SumI2OutMin=[]  SumI2OutMax=[]  SumI3OutMin=[]  SumI3OutMax=[]  SumI4OutMin=[]  SumI4OutMax=[]  SumDOutMin=[]  SumDOutMax=[]  DifferentiatorOutMin=[]  DifferentiatorOutMax=[]  FilterDiffOutCoefMin=[]  FilterDiffOutCoefMax=[]  ReciprocalOutMin=[]  ReciprocalOutMax=[]  SumDenOutMin=[]  SumDenOutMax=[]  SumNumOutMin=[]  SumNumOutMax=[]  DivideOutMin=[]  DivideOutMax=[]  UdiffTsProdOutMin=[]  UdiffTsProdOutMax=[]  NTsProdOutMin=[]  NTsProdOutMax=[]  UintegralTsProdOutMin=[]  UintegralTsProdOutMax=[]  UngainTsProdOutMin=[]  UngainTsProdOutMax=[]  ClampingZeroOutDataTypeStr=Inherit: Inherit via back propagation  ClampingZeroOutMin=[]  ClampingZeroOutMax=[]  FilterDenConstantOutDataTypeStr=Inherit: Inherit via back propagation  FilterDenConstantOutMin=[]  FilterDenConstantOutMax=[]  PCopyOutDataTypeStr=Inherit: Inherit via back propagation  PCopyOutMin=[]  PCopyOutMax=[]  NCopyOutDataTypeStr=Inherit: Inherit via back propagation  NCopyOutMin=[]  NCopyOutMax=[]  IntegratorContinuousStateAttributes=''  IntegratorStateMustResolveToSignalObject=off  IntegratorRTWStateStorageClass=Auto  FilterContinuousStateAttributes=''  FilterStateMustResolveToSignalObject=off  FilterRTWStateStorageClass=Auto  ParallelPVariant=InternalParameters  IdealPVariant=Disabled  IVariant=InternalParameters  DVariant=InternalParameters  IntegratorVariant=Continuous  SatVariant=Disabled  AWVariant=Passthrough  PCopyVariant=Disabled  TRVariant=Disabled  FdbkBlocksVariant=Forward  IdealPFdbkVariant=Disabled  SatFdbkVariant=Disabled  DerivativeFilterVariant=ContFilter  NVariant=InternalParameters  NCopyVariant=Disabled  FilterICVariant=InternalICsFilter  IntegratorICVariant=InternalICs  ExternalResetVariant=Disabled  TRSumVariant=Passthrough  SumFdbkVariant=Disabled  SumVariant=Sum_PID  TsampFilterVariant=InternalTs  TsampNgainVariant=Passthrough  TsampIntegralVariant=Disabled_SignalSpec  ExternalSaturationOutDataTypeStr=Inherit: Same as second input
  Pulse Generator : DiscretePulseGenerator  PulseType=Time based  Amplitude=5  Period=40  PulseWidth=50
  Scope{,1..7} (8 alike) : Scope
  Step : Step  Time=20  After=5  SampleTime=0
  Sum{1..9} (9 alike) : Sum  Inputs=|+-
  Sum{10..13} (4 alike) : Sum  Inputs=|++
  Terminator{1,5..8} (5 alike) : Terminator
  Out1 : Outport
  wires:
  Constant1/1 -> Sum9/2, Sum9/1
  [teteeksifo] -> Sum11/2
  PID Controller10/1 -> [teteeksifo]
  [tetefo] -> Sum10/2
  PID Controller9/1 -> [tetefo]
  Sum9/1 -> PID Controller9/1, PID Controller10/1
  Sum11/1 -> Mux/6
  PID Controller2/1 -> Sum11/1
  Sum10/1 -> Mux/5
  PID Controller1/1 -> Sum10/1
  Sum4/1 -> PID Controller4/1
  Sum3/1 -> PID Controller3/1
  Sum2/1 -> PID Controller2/1
  Sum1/1 -> PID Controller1/1
  [xyon] -> Sum8/1
  [xyon] -> Sum6/1
  [xyon] -> Sum5/1
  [xyon] -> Sum7/1
  Sum8/1 -> PID Controller8/1
  PID Controller8/1 -> Mux/4
  PID Controller7/1 -> Mux/2
  Sum7/1 -> PID Controller7/1
  PID Controller6/1 -> Mux/3
  Sum6/1 -> PID Controller6/1
  PID Controller5/1 -> Mux/1
  Sum5/1 -> PID Controller5/1
  Mux1/1 -> Scope1/1
  Demux1/4 -> Terminator8/1
  Demux1/8 -> Mux1/4
  Demux1/7 -> Mux1/3
  Demux1/5 -> Mux1/1
  Demux1/6 -> Mux1/2
  Demux1/3 -> Terminator7/1
  Demux1/2 -> Terminator6/1
  Demux1/1 -> Terminator5/1
  Demux/3 -> Sum1/2, Scope/1, Sum2/2, Sum3/2, Sum4/2
  Demux/4 -> Scope4/1
  Demux/5 -> Scope5/1, [teta]
  Demux/6 -> Scope6/1
  Demux/2 -> Scope3/1
  Demux/1 -> [xval], Scope2/1
  Input/1 -> Demux/1
  Mux/1 -> Out1/1, Demux1/1
  Constant4/1 -> Sum4/1
  Constant3/1 -> Sum3/1
  Constant2/1 -> Sum2/1
  Constant/1 -> Sum1/1
  [xval] -> Sum5/2
  [xval] -> Sum7/2
  [xval] -> Sum6/2
  [xval] -> Sum8/2
  Sum12/1 -> Mux/7
  Sum13/1 -> Mux/8
  PID Controller3/1 -> Sum12/1
  PID Controller4/1 -> Sum13/1
  [tetefo] -> Sum13/2
  [teteeksifo] -> Sum12/2
  Pulse Generator/1 -> [xyon], Scope7/1
  Step/1 -> Terminator1/1

== matlab function dinamicaralik/Subsystem/CA/MATLAB Function ==
  data: Vw input; y output
function y = fcn(Vw)

u = Vw(1);
v = Vw(2);
w = Vw(3);

p = Vw(4);
q = Vw(5);
r = Vw(6);

Xu_dot = -5.5;   % Surge direction
Yv_dot = -12.7;  % Sway direction
Zw_dot = -14.57; % Heave direction

Kp_dot = -0.12;  % Roll moment
Mq_dot = -0.12;  % Pitch moment
Nr_dot = -0.12;  % Yaw moment



% ek kütle corriolis Matrisin tanımlanması
    CA = [
        0,        0,          0,        0,          Zw_dot*w,  0        ;
        0,        0,          0,       -Zw_dot*w,   0,         -Xu_dot*u;
        0,        0,          0,       -Yv_dot*v,   Xu_dot*u,  0        ;
        0,       -Zw_dot*w,  Yv_dot*v,  0,         -Nr_dot*r,  Mq_dot*q ;
        Zw_dot*w, 0,        -Xu_dot*u,  Nr_dot*r,   0,        -Kp_dot*p ;
       -Yv_dot*v, Xu_dot*u,   0,       -Mq_dot*q,   Kp_dot*p,  0        ;
    ];


y = CA * Vw ;

== matlab function dinamicaralik/pwm to fource/MATLAB Function1 ==
  data: u input; y output
function y = Normalize(u)
y = (u-1500)*150/400;

== matlab function dinamicaralik/pwm to fource/MATLAB Function2 ==
  data: u input; y output
function y = Normalize(u)
y = (u-1500)*150/400;

== matlab function dinamicaralik/pwm to fource/MATLAB Function3 ==
  data: u input; y output
function y = Normalize(u)
y = (u-1500)*150/400;

== matlab function dinamicaralik/pwm to fource/MATLAB Function4 ==
  data: u input; y output
function y = Normalize(u)
y = (u-1500)*150/400;

== matlab function dinamicaralik/pwm to fource/MATLAB Function5 ==
  data: u input; y output
function y = Normalize(u)
y = (u-1500)*150/400;

== matlab function dinamicaralik/pwm to fource/MATLAB Function6 ==
  data: u input; y output
function y = Normalize(u)
y = (u-1500)*150/400;

== matlab function dinamicaralik/pwm to fource/MATLAB Function7 ==
  data: u input; y output
function y = Normalize(u)
y = (u-1500)*150/400;

== matlab function dinamicaralik/Subsystem/MA/MATLAB Function ==
  data: accelW input; y output
function y = fcn(accelW)
% Add mass parametreleri
Xu_dot = -5.5;   % Surge direction
Yv_dot = -12.7;  % Sway direction
Zw_dot = -14.57; % Heave direction

Kp_dot = -0.12;  % Roll moment
Mq_dot = -0.12;  % Pitch moment
Nr_dot = -0.12;  % Yaw moment

% MA Matrisinin tanımlanması
MA = -[
        Xu_dot,    0,       0,       0,       0,       0;
        0,       Yv_dot,    0,       0,       0,       0;
        0,         0,     Zw_dot,    0,       0,       0;
        0,         0,       0,     Kp_dot,   0,       0;
        0,         0,       0,       0,     Mq_dot,   0;
        0,         0,       0,       0,       0,     Nr_dot
    ];

y = MA * accelW;

== matlab function dinamicaralik/Subsystem1/MATLAB Function10 ==
  data: F3 input; thrust3 output
function thrust3 = fcn(F3)

% T3
lx3 = -156 / 1000; % metre
ly3 = 111 / 1000;  % metre
lz3 = 85 / 1000;   % metre
F3q = pi/4;


Fx = -F3 * cos(F3q);
Fy = -F3 * sin(F3q);
Fz = 0;

% Matrisin tanımlanması
forces_and_moments = [
    Fx;                  % Kuvvet: x bileşeni
    Fy;                  % Kuvvet: y bileşeni
    Fz;                  % Kuvvet: z bileşeni
    Fz*ly3 - Fy*lz3;    % Moment: x ekseni etrafında
    Fx*lz3 - Fz*lx3;    % Moment: y ekseni etrafında
    (Fy*lx3 - Fx*ly3)     % Moment: z ekseni etrafında burda da bi fark var
];
% Sonuçların görüntülenmesi
%disp('Forces and Moments Matrix:');
%disp(forces_and_moments);

thrust3 = forces_and_moments;

== matlab function dinamicaralik/Subsystem1/MATLAB Function11 ==
  data: F4 input; thrust4 output
function thrust4 = fcn(F4)

% T4
lx4 = -156 / 1000; % metre
ly4 = -111 / 1000; % metre
lz4 = 85 / 1000;   % metre
F4q = pi/4;

Fx = -F4 * cos(F4q);
Fy = F4 * sin(F4q);
Fz = 0;

% Matrisin tanımlanması
forces_and_moments = [
    Fx;                  % Kuvvet: x bileşeni
    Fy;                  % Kuvvet: y bileşeni
    Fz;                  % Kuvvet: z bileşeni
    Fz*ly4 - Fy*lz4;    % Moment: x ekseni etrafında
    Fx*lz4 - Fz*lx4;    % Moment: y ekseni etrafında
    (Fy*lx4 - Fx*ly4)     % Moment: z ekseni etrafında bu da farkli
];
% Sonuçların görüntülenmesi
%disp('Forces and Moments Matrix:');
%disp(forces_and_moments);

thrust4 = forces_and_moments;

== matlab function dinamicaralik/Subsystem/inv MA and MRB/MRB sadece ==
  data: u input; y output
function y = fcn(u)

m = 10.5     ;  % aracın kütlesi kg

xg = 0 ; % rgid body frame e göre ağırlık merkzi kordinatları
yg = 0 ;
zg = 0.02 ;

Ix = 0.1011 ; % kg *  m ^2 
Iy = 0.1159 ;
Iz = 0.1615 ;


% MRB Matrisinin tanımlanması
MRB = [
        m,    0,    0,    0,   m*zg,  0;
        0,    m,    0, -m*zg,   0,    0;
        0,    0,    m,    0,    0,    0;
        0, -m*zg,   0,   Ix,    0,    0;
       m*zg,  0,    0,    0,   Iy,    0;
        0,    0,    0,    0,    0,   Iz
    ];


y = (MRB) \ u ; % M_product * y = u denkleminden y'i çözer

== matlab function dinamicaralik/Subsystem1/MATLAB Function12 ==
  data: F5 input; thrust5 output
function thrust5 = fcn(F5)

% T5
lx5 = 120 / 1000;  % metre
ly5 = 218 / 1000;  % metre
lz5 = 0 / 1000;    % metre

Fx = 0*F5;
Fy = 0*F5;
Fz = -1*F5;

% Matrisin tanımlanması
forces_and_moments = [
    Fx;                  % Kuvvet: x bileşeni
    Fy;                  % Kuvvet: y bileşeni
    Fz;                  % Kuvvet: z bileşeni
    Fz*ly5 - Fy*lz5;    % Moment: x ekseni etrafında
    Fx*lz5 - Fz*lx5;    % Moment: y ekseni etrafında
    Fy*lx5 - Fx*ly5     % Moment: z ekseni etrafında
];


thrust5 = forces_and_moments;

== matlab function dinamicaralik/Subsystem1/MATLAB Function13 ==
  data: F6 input; thrust6 output
function thrust6 = fcn(F6)


% T6
lx6 = 120 / 1000;  % metre
ly6 = -218 / 1000; % metre
lz6 = 0 / 1000;    % metre


Fx = 0*F6;
Fy = 0*F6;
Fz = 1*F6;

% Matrisin tanımlanması
forces_and_moments = [
    Fx;                  % Kuvvet: x bileşeni
    Fy;                  % Kuvvet: y bileşeni
    Fz;                  % Kuvvet: z bileşeni
    Fz*ly6 - Fy*lz6;    % Moment: x ekseni etrafında
    Fx*lz6 - Fz*lx6;    % Moment: y ekseni etrafında
    Fy*lx6 - Fx*ly6     % Moment: z ekseni etrafında
];
% Sonuçların görüntülenmesi
%disp('Forces and Moments Matrix:');
%disp(forces_and_moments);

thrust6 = forces_and_moments;

== matlab function dinamicaralik/Subsystem1/MATLAB Function14 ==
  data: F7 input; thrust7 output
function thrust7 = fcn(F7)

% T7
lx7 = -120 / 1000; % metre
ly7 = 218 / 1000;  % metre
lz7 = 0 / 1000;    % metre

Fx = 0*F7;
Fy = 0*F7;
Fz = 1*F7;

% Matrisin tanımlanması
forces_and_moments = [
    Fx;                  % Kuvvet: x bileşeni
    Fy;                  % Kuvvet: y bileşeni
    Fz;                  % Kuvvet: z bileşeni
    Fz*ly7 - Fy*lz7;    % Moment: x ekseni etrafında
    Fx*lz7 - Fz*lx7;    % Moment: y ekseni etrafında
    Fy*lx7 - Fx*ly7     % Moment: z ekseni etrafında
];
% Sonuçların görüntülenmesi
disp('Forces and Moments Matrix:');
disp(forces_and_moments);

thrust7 = forces_and_moments;

== matlab function dinamicaralik/Subsystem1/MATLAB Function15 ==
  data: F8 input; thrust8 output
function thrust8 = fcn(F8)

% T8
lx8 = -120 / 1000; % metre
ly8 = -218 / 1000; % metre
lz8 = 0 / 1000;    % metre

Fx = 0*F8;
Fy = 0*F8;
Fz = -1*F8;

% Matrisin tanımlanması
forces_and_moments = [
    Fx;                  % Kuvvet: x bileşeni
    Fy;                  % Kuvvet: y bileşeni
    Fz;                  % Kuvvet: z bileşeni
    Fz*ly8 - Fy*lz8;    % Moment: x ekseni etrafında
    Fx*lz8 - Fz*lx8;    % Moment: y ekseni etrafında
    Fy*lx8 - Fx*ly8     % Moment: z ekseni etrafında
];
% Sonuçların görüntülenmesi
disp('Forces and Moments Matrix:');
disp(forces_and_moments);

thrust8 = forces_and_moments;

== matlab function dinamicaralik/Subsystem1/MATLAB Function8 ==
  data: F1 input; thrust1 output
function thrust1 = fcn(F1)

% T1
lx1 = 156 / 1000;  % metre
ly1 = 111 / 1000;  % metre
lz1 = 85 / 1000;   % metre
F1q = pi/4;

Fx = F1 * cos(F1q);
Fy = -F1 * sin(F1q);
Fz = 0;

% Matrisin tanımlanması
forces_and_moments = [
    Fx;                  % Kuvvet: x bileşeni
    Fy;                  % Kuvvet: y bileşeni
    Fz;                  % Kuvvet: z bileşeni
    Fz*ly1 - Fy*lz1;    % Moment: x ekseni etrafında
    Fx*lz1 - Fz*lx1;    % Moment: y ekseni etrafında
    Fy*lx1 - Fx*ly1     % Moment: z ekseni etrafında
];
% Sonuçların görüntülenmesi
%disp('Forces and Moments Matrix:');
%disp(forces_and_moments);

thrust1 = forces_and_moments;

== matlab function dinamicaralik/Subsystem1/MATLAB Function9 ==
  data: F2 input; thrust2 output
function thrust2 = fcn(F2)

% T2
lx2 = 156 / 1000;  % metre
ly2 = -111 / 1000; % metre
lz2 = 85 / 1000;   % metre
F2q = pi/4;

Fx = F2 * cos(F2q);
Fy = F2 * sin(F2q);
Fz = 0;

% Matrisin tanımlanması
forces_and_moments = [
    Fx;                  % Kuvvet: x bileşeni
    Fy;                  % Kuvvet: y bileşeni
    Fz;                  % Kuvvet: z bileşeni
    Fz*ly2 - Fy*lz2;    % Moment: x ekseni etrafında
    Fx*lz2 - Fz*lx2;    % Moment: y ekseni etrafında
    (Fy*lx2 - Fx*ly2)     % Moment: z ekseni etrafında burda liva farklı yapmıs
];
% Sonuçların görüntülenmesi
%disp('Forces and Moments Matrix:');
%disp(forces_and_moments);

thrust2 = forces_and_moments;

== matlab function dinamicaralik/Body to euler/euler transform ==
  data: veloB input; NEDvelo output
function NEDvelo = fcn(veloB)

phi = pi;

theta = 0;

psi = 0;

Rbn = [
    cos(psi)*cos(theta), -sin(psi)*cos(phi) + cos(psi)*sin(theta)*sin(phi),  sin(psi)*sin(phi) + cos(psi)*cos(phi)*sin(theta);
    sin(psi)*cos(theta),  cos(psi)*cos(phi) + sin(psi)*sin(theta)*sin(phi), -cos(psi)*sin(phi) + sin(psi)*cos(phi)*sin(theta);
   -sin(theta),          cos(theta)*sin(phi),                              cos(theta)*cos(phi)
];


Ttheta = [
    1, sin(phi)*tan(theta), cos(phi)*tan(theta);
    0, cos(phi),           -sin(phi);
    0, sin(phi)/cos(theta), cos(phi)/cos(theta)
];

% 0_3x3 sıfır matrisi
Zero3x3 = zeros(3);

% Jacobian matrisi J_Theta(eta)
JTheta = [
    Rbn,      Zero3x3;
    Zero3x3,  Ttheta
];


NEDvelo = JTheta * veloB;

== matlab function dinamicaralik/Subsystem/inv MA and MRB/MA ve MRB ==
  data: u input; y output
function y = fcn(u)

m = 10.5     ;  % aracın kütlesi kg

xg = 0 ; % rgid body frame e göre ağırlık merkzi kordinatları
yg = 0 ;
zg = 0.02;

Ix = 0.1011 ; % kg *  m ^2 
Iy = 0.1159 ;
Iz = 0.1615 ;


% MRB Matrisinin tanımlanması
MRB = [
        m,    0,    0,    0,   m*zg,  0;
        0,    m,    0, -m*zg,   0,    0;
        0,    0,    m,    0,    0,    0;
        0, -m*zg,   0,   Ix,    0,    0;
       m*zg,  0,    0,    0,   Iy,    0;
        0,    0,    0,    0,    0,   Iz
    ];


Xu_dot = -5.5;   % Surge direction
Yv_dot = -12.7;  % Sway direction
Zw_dot = -14.57; % Heave direction

Kp_dot = -0.12;  % Roll moment
Mq_dot = -0.12;  % Pitch moment
Nr_dot = -0.12;  % Yaw moment

% MA Matrisinin tanımlanması
MA = -[
        Xu_dot,    0,       0,       0,       0,       0;
        0,       Yv_dot,    0,       0,       0,       0;
        0,         0,     Zw_dot,    0,       0,       0;
        0,         0,       0,     Kp_dot,   0,       0;
        0,         0,       0,       0,     Mq_dot,   0;
        0,         0,       0,       0,       0,     Nr_dot
    ];

%inv([m 0 0 0 0 0;0 m 0 0 0 0;0 0 m 0 0 0;0 0 0 Ix 0 0;0 0 0 0 Iy 0;0 0 0 0 0 Iz]+[Xudot 0 0 0 0 0;0 Yvdot 0 0 0 0;0 0 Zwdot 0 0 0;0 0 0 Kpdot 0 0;0 0 0 0 Mqdot 0;0 0 0 0 0 Nrdot])
y = inv(MRB + MA) * u ; % M_product * y = u denkleminden y'i çözer

== matlab function dinamicaralik/Body to euler1/euler transform ==
  data: veloB input; NEDvelo output
function NEDvelo = fcn(veloB)

phi = pi;

theta = 0;

psi = 0;

Rbn = [
    cos(psi)*cos(theta), -sin(psi)*cos(phi) + cos(psi)*sin(theta)*sin(phi),  sin(psi)*sin(phi) + cos(psi)*cos(phi)*sin(theta);
    sin(psi)*cos(theta),  cos(psi)*cos(phi) + sin(psi)*sin(theta)*sin(phi), -cos(psi)*sin(phi) + sin(psi)*cos(phi)*sin(theta);
   -sin(theta),          cos(theta)*sin(phi),                              cos(theta)*cos(phi)
];


Ttheta = [
    1, sin(phi)*tan(theta), cos(phi)*tan(theta);
    0, cos(phi),           -sin(phi);
    0, sin(phi)/cos(theta), cos(phi)/cos(theta)
];

% 0_3x3 sıfır matrisi
Zero3x3 = zeros(3);

% Jacobian matrisi J_Theta(eta)
JTheta = [
    Rbn,      Zero3x3;
    Zero3x3,  Ttheta
];


NEDvelo = JTheta * veloB;

== matlab function dinamicaralik/Subsystem3/CA/MATLAB Function ==
  data: Vw input; y output
function y = fcn(Vw)

u = Vw(1);
v = Vw(2);
w = Vw(3);

p = Vw(4);
q = Vw(5);
r = Vw(6);

Xu_dot = -5.5;   % Surge direction
Yv_dot = -12.7;  % Sway direction
Zw_dot = -14.57; % Heave direction

Kp_dot = -0.12;  % Roll moment
Mq_dot = -0.12;  % Pitch moment
Nr_dot = -0.12;  % Yaw moment



% ek kütle corriolis Matrisin tanımlanması
    CA = [
        0,        0,          0,        0,          Zw_dot*w,  0        ;
        0,        0,          0,       -Zw_dot*w,   0,         -Xu_dot*u;
        0,        0,          0,       -Yv_dot*v,   Xu_dot*u,  0        ;
        0,       -Zw_dot*w,  Yv_dot*v,  0,         -Nr_dot*r,  Mq_dot*q ;
        Zw_dot*w, 0,        -Xu_dot*u,  Nr_dot*r,   0,        -Kp_dot*p ;
       -Yv_dot*v, Xu_dot*u,   0,       -Mq_dot*q,   Kp_dot*p,  0        ;
    ];


y = CA * Vw ;

== matlab function dinamicaralik/Subsystem/CRB/MATLAB Function ==
  data: V input; y output
function y = fcn(V)

u = V(1);
v = V(2);
w = V(3);

p = V(4);
q = V(5);
r = V(6);

Ix = 0.1011 ; % kg *  m ^2 
Iy = 0.1159 ;
Iz = 0.1615 ;

m = 10.5     ;  % aracın kütlesi kg

% Matrisin tanımlanması
CRB = [
        0,     0,     0,        0,   m*w,    0;
        0,     0,     0,     -m*w,     0,    0;
        0,     0,     0,      m*v,  -m*u,    0;
        0,     m*w,  -m*v,    0,     Iz*r,  -Iy*q;
        -m*w,  0,    -m*u,   -Iz*r,    0,    Ix*p;
        m*v,  -m*u,   0,      Iy*q, -Ix*p,   0;
    ];

y= CRB * V ;
